simulink model "mymodel"  (R2024a)
settings: Solver=VariableStepAuto  StartTime=0.0  StopTime=10.0  RelTol=1e-3
settings Model: Creator=Wyatt  LastModifiedBy=Wyatt

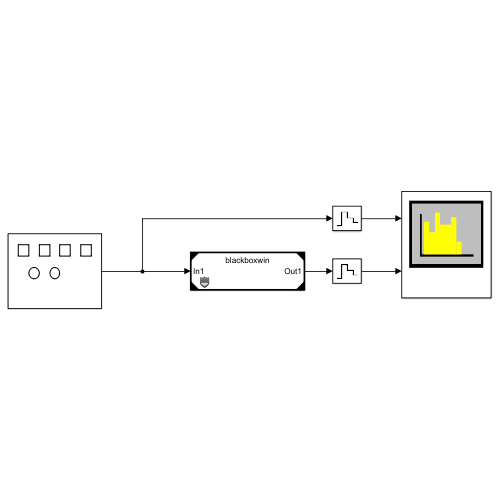
[thumbnail: Simulink's stored preview of the top-level diagram]
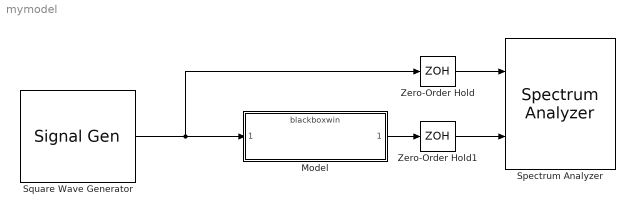
== system mymodel ==
  Model : ModelReference  ModelNameDialog=blackboxwin.slxp  ModelReferenceVersion=1.1  CopyOfModelProtected=on
  Spectrum Analyzer : SpectrumAnalyzer  NumInputPorts=2  WindowPosition=[0.000000,36.000000,1536.000000,792.000000,]  Visible=on  ScopeFrameLocation=window  Method=Welch  PlotAsTwoSidedSpectrum=off  FrequencyResolutionMethod=Window length  WindowLength=10000  Span=49999.99999999999  CenterFrequency=24999.999999999996  StartFrequency=0  StopFrequency=49999.99999999999  Window=Flat Top  YLimits=[-397.77269563,76.51686172]
  Square Wave Generator : SignalGenerator  WaveForm=square
  Zero-Order Hold : ZeroOrderHold  SampleTime=1/(2e3)
  Zero-Order Hold1 : ZeroOrderHold  SampleTime=1/(2e3)
  wires:
  Square Wave Generator/1 -> Zero-Order Hold/1, Model/1
  Model/1 -> Zero-Order Hold1/1
  Zero-Order Hold1/1 -> Spectrum Analyzer/2
  Zero-Order Hold/1 -> Spectrum Analyzer/1
